simulink model "p1_MCU"  (R2023a)
settings: Solver=FixedStepDiscrete  StartTime=0.0  StopTime=inf  FixedStep=Ts_MCU  RelTol=1e-3  EnableMultiTasking=on
PreLoadFcn:
  | p1_params_new
  | spiDataDefinition
InitFcn:
  | mbd_s32k_consistency_checks(bdroot(gcs));
undefined symbols (not defined in the file or in its folder): ack, cpr_handwheel, cpr_steering, Discrete, DriverInput, DrivetrainLeft, DrivetrainRight, LQFP, MPU_IO, n_handwheel, n_steering, p1data, p1params, param, sr, steering_limit, SteeringLeft, SteeringRight, Time, Ts_MCU, wc, WheelForceLeft, WheelForceRight
libraries: simulink x74, mbd_s32k1xx_ec_toolbox x58, Library_Drivetrain x5, Library_Steering x5, etargetslib x3, ctrlSharedLib x1
(part 2 of 4)

== system p1_MCU/Subsystem ==
  ADC_Config : mbd_s32k1xx_ec_toolbox/Motor Control Blocks/ADC Blocks/ADC_Config  instance=0  mode=12-bit conversion  smplts=20  adiclk=alternate clock 1  adiv=input clock  show_adv_opts=on  pretrgsel=PDB pre-trigger  swpretrg=Disabled  adtrg=software  trgsel=TRGMUX output  refsel=Vrefh and Vrefl  supply_monitoring=off  acfe=off  acfgt=off  acren=off  cv1=0  cv2=0  adco=off  avge=off  avgs=4 samples
  ADC_Config1 : mbd_s32k1xx_ec_toolbox/Motor Control Blocks/ADC Blocks/ADC_Config  instance=1  mode=12-bit conversion  smplts=20  adiclk=alternate clock 1  adiv=input clock  show_adv_opts=on  pretrgsel=PDB pre-trigger  swpretrg=Disabled  adtrg=software  trgsel=TRGMUX output  refsel=Vrefh and Vrefl  supply_monitoring=off  acfe=off  acfgt=off  acren=off  cv1=0  cv2=0  adco=off  avge=off  avgs=4 samples
  Init Processor : mbd_s32k1xx_ec_toolbox/MBD_S32K1xx_Config_Information  mbdt_ver=0  disp_str=|  config_params=[]  mcu_target_name=S32K144  mcu_target_package=100-LQFP  mcu_target_sram_size=64KB  mcu_system_clock_freq=80  mcu_xtal_freq=External 8  mcu_steptick_timer=LPIT Channel 0  mcu_steptick_prio=15  ds_import_enable=on  target_compiler=GCC  target_memory=FLASH  gcc_target_compile_opts=-mcpu=cortex-m4 -mthumb -mfloat-abi=hard -mfpu=fpv4-sp-d16 -O1 -g -gstrict-dwarf  gcc_target_assemble_opts=-mcpu=cortex-m4 -mthumb -mfloat-abi=hard -mfpu=fpv4-sp-d16 -g  gcc_target_link_opts=-mcpu=cortex-m4 -mthumb -mfloat-abi=hard -mfpu=fpv4-sp-d16  gcc_target_default_lcf=on  gcc_target_user_lcf=S32K148_192_flash.ld  ghs_target_compile_opts=-cpu=cortexm4f -thumb -DARM_MATH_CM4 -fpu=vfpv4_d16 -fsingle -Ogeneral -Wundef -Wimplicit-int -Wshadow -Wtrigraphs --no_commons --gnu_asm -gnu99 -gdwarf-2 -G  ghs_target_assemble_opts=-cpu=cortexm4f -fpu=vfpv4_d16  ghs_target_link_opts=-cpu=cortexm4f -thumb -fpu=vfpv4_d16  ghs_target_default_lcf=on  ghs_target_user_lcf=S32K148_192_flash.ld  iar_target_compile_opts=--cpu=Cortex-M4F --thumb --fpu=VFPv4_sp -Ol -e --debug --dlib_config normal  iar_target_assemble_opts=--cpu Cortex-M4F --thumb --fpu VFPv4_sp  iar_target_link_opts=--no_exceptions --vfe --inline  iar_target_default_lcf=on  iar_target_user_lcf=S32K148_192_flash.icf  pil_download_enable=off  rbl_download_enable=off  rbl_start_delay=5000000  rbl_download_interface=OpenSDA  rbl_restart_request=off  rbl_com_port=Custom  rbl_com_port_custom=COM1  pil_download_rate=57600  pil_opensda_drive=Custom  pil_opensda_drive_custom=D  pil_uart_instance=1  pil_uart_rx=PTC6: [LPUART1_RX | Receive]  pil_uart_tx=PTC7: [LPUART1_TX | Transmit]  FTM_PWM_PcrCheckEnDis=on  FTM_Input_Edge_Inputs_PcrCheckEnDis=on  FTM_Dual_Edge_Inputs_PcrCheckEnDis=on  FTM_Quadrature_Inputs_PcrCheckEnDis=on  FTM_Hall_Sensor_Inputs_PcrCheckEnDis=on  LPTMR_PcrCheckEnDis=on  PIT_PcrCheckEnDis=on  RTC_PcrCheckEnDis=on  FlexCAN_PcrCheckEnDis=on  LIN_PcrCheckEnDis=on  FlexIO_PcrCheckEnDis=on  LPI2C_PcrCheckEnDis=on  LPSPI_PcrCheckEnDis=on  LPUART_PcrCheckEnDis=on  CMP_PcrCheckEnDis=on  GPIO_OutputPcrCheckEnDis=on  GPIO_InputPcrCheckEnDis=on  SBC_PcrCheckEnDis=on  BMS_PcrCheckEnDis=on  AMMCLIB_PcrCheckEnDis=on  FM_PcrCheckEnDis=on  Profile_PcrCheckEnDis=on  ConfigParams_PcrCheckEnDis=on  ModelRef_PcrCheckEnDis=on  PDB0_PcrCheckEnDis=on  CSEc_PcrCheckEnDis=on  eDMA_PcrCheckEnDis=on  FLASH_PcrCheckEnDis=on  ADC_PcrCheckEnDis=on  WDOG_PcrCheckEnDis=on
      | Target : S32K144-64KB_SRAM
      | Package : 100-pin
      | System clock : 80 MHz
      | XTAL clock : External 8 MHz
      | Compiler : IAR
      | Target Type : FLASH
      | Download Code after build : off
      | Step Tick Interrupt Priority : 15
  Init_CAN0_500kbit : mbd_s32k1xx_ec_toolbox/Communication Blocks/CAN Blocks/FCAN_Config  Priority=1  can_instance=0  can_mode=Normal mode  can_max_num_mb=16  can_rx=PTB0: [CAN0_RX | CAN Rx channel]  can_tx=PTB1: [CAN0_TX | CAN Tx Channel]  show_adv_opts=off  can_clk_src=Peripheral clock  bitrate=500  bitrate_adv_opts=off  can_presdiv=7  can_rjw=3  can_pseg1=6  can_pseg2=3  can_propseg=7  can_cbt_presdiv=9  can_cbt_rjw=0  can_cbt_pseg1=3  can_cbt_pseg2=3  can_cbt_propseg=6  can_fd_enable=off  can_payload=8  can_rxfifo_enable=off  can_fifo_id_filter_extended=off  can_fifo_id_filter_remote=off  can_num_id_filters=8  can_fifo_id_format=A  can_fifo_id_filter={'0x0', '0x0', '0x0', '0x0', '0x0', '0x0', '0x0', '0x0'}  can_pn_enable=off  can_wakeup_match=off  can_wakeup_timeout=off  can_timeout_en=off  can_match_timeout=1  can_multiple_matches_en=off  can_num_matches=1  can_idfilter_extendedid=off  can_idfilter_remoteframe=off  can_idfilter_type=Match exact  can_idfilter_id1=0  can_idfilter_id2=0  can_payloadfilter_enable=on  can_payloadfilter_dlclow=0  can_payloadfilter_dlchigh=0  can_payloadfilter_type=Match exact  can_payloadfilter_payload1_b0=0  can_payloadfilter_payload1_b1=0  can_payloadfilter_payload1_b2=0  can_payloadfilter_payload1_b3=0  can_payloadfilter_payload1_b4=0  can_payloadfilter_payload1_b5=0  can_payloadfilter_payload1_b6=0  can_payloadfilter_payload1_b7=0  can_payloadfilter_payload2_b0=0  can_payloadfilter_payload2_b1=0  can_payloadfilter_payload2_b2=0  can_payloadfilter_payload2_b3=0  can_payloadfilter_payload2_b4=0  can_payloadfilter_payload2_b5=0  can_payloadfilter_payload2_b6=0  can_payloadfilter_payload2_b7=0
  Init_CAN1_500kbit1 : mbd_s32k1xx_ec_toolbox/Communication Blocks/CAN Blocks/FCAN_Config  Priority=1  can_instance=1  can_mode=Normal mode  can_max_num_mb=16  can_rx=PTA12: [CAN1_RX | CAN Rx channel]  can_tx=PTA13: [CAN1_TX | CAN Tx Channel]  show_adv_opts=off  can_clk_src=Peripheral clock  bitrate=500  bitrate_adv_opts=off  can_presdiv=7  can_rjw=3  can_pseg1=6  can_pseg2=3  can_propseg=7  can_cbt_presdiv=9  can_cbt_rjw=0  can_cbt_pseg1=3  can_cbt_pseg2=3  can_cbt_propseg=6  can_fd_enable=off  can_payload=8  can_rxfifo_enable=off  can_fifo_id_filter_extended=off  can_fifo_id_filter_remote=off  can_num_id_filters=8  can_fifo_id_format=A  can_fifo_id_filter={'0x0', '0x0', '0x0', '0x0', '0x0', '0x0', '0x0', '0x0'}  can_pn_enable=off  can_wakeup_match=off  can_wakeup_timeout=off  can_timeout_en=off  can_match_timeout=1  can_multiple_matches_en=off  can_num_matches=1  can_idfilter_extendedid=off  can_idfilter_remoteframe=off  can_idfilter_type=Match exact  can_idfilter_id1=0  can_idfilter_id2=0  can_payloadfilter_enable=on  can_payloadfilter_dlclow=0  can_payloadfilter_dlchigh=0  can_payloadfilter_type=Match exact  can_payloadfilter_payload1_b0=0  can_payloadfilter_payload1_b1=0  can_payloadfilter_payload1_b2=0  can_payloadfilter_payload1_b3=0  can_payloadfilter_payload1_b4=0  can_payloadfilter_payload1_b5=0  can_payloadfilter_payload1_b6=0  can_payloadfilter_payload1_b7=0  can_payloadfilter_payload2_b0=0  can_payloadfilter_payload2_b1=0  can_payloadfilter_payload2_b2=0  can_payloadfilter_payload2_b3=0  can_payloadfilter_payload2_b4=0  can_payloadfilter_payload2_b5=0  can_payloadfilter_payload2_b6=0  can_payloadfilter_payload2_b7=0
  Init_CAN1_500kbit2 : mbd_s32k1xx_ec_toolbox/Communication Blocks/CAN Blocks/FCAN_Config  Priority=1  can_instance=2  can_mode=Normal mode  can_max_num_mb=16  can_rx=PTC16: [CAN2_RX | CAN Rx channel]  can_tx=PTC17: [CAN2_TX | CAN Tx Channel]  show_adv_opts=off  can_clk_src=Peripheral clock  bitrate=500  bitrate_adv_opts=off  can_presdiv=7  can_rjw=3  can_pseg1=6  can_pseg2=3  can_propseg=7  can_cbt_presdiv=9  can_cbt_rjw=0  can_cbt_pseg1=3  can_cbt_pseg2=3  can_cbt_propseg=6  can_fd_enable=off  can_payload=8  can_rxfifo_enable=off  can_fifo_id_filter_extended=off  can_fifo_id_filter_remote=off  can_num_id_filters=8  can_fifo_id_format=A  can_fifo_id_filter={'0x0', '0x0', '0x0', '0x0', '0x0', '0x0', '0x0', '0x0'}  can_pn_enable=off  can_wakeup_match=off  can_wakeup_timeout=off  can_timeout_en=off  can_match_timeout=1  can_multiple_matches_en=off  can_num_matches=1  can_idfilter_extendedid=off  can_idfilter_remoteframe=off  can_idfilter_type=Match exact  can_idfilter_id1=0  can_idfilter_id2=0  can_payloadfilter_enable=on  can_payloadfilter_dlclow=0  can_payloadfilter_dlchigh=0  can_payloadfilter_type=Match exact  can_payloadfilter_payload1_b0=0  can_payloadfilter_payload1_b1=0  can_payloadfilter_payload1_b2=0  can_payloadfilter_payload1_b3=0  can_payloadfilter_payload1_b4=0  can_payloadfilter_payload1_b5=0  can_payloadfilter_payload1_b6=0  can_payloadfilter_payload1_b7=0  can_payloadfilter_payload2_b0=0  can_payloadfilter_payload2_b1=0  can_payloadfilter_payload2_b2=0  can_payloadfilter_payload2_b3=0  can_payloadfilter_payload2_b4=0  can_payloadfilter_payload2_b5=0  can_payloadfilter_payload2_b6=0  can_payloadfilter_payload2_b7=0
  "LPSPI_Config " : mbd_s32k1xx_ec_toolbox/Communication Blocks/SPI Blocks/LPSPI_Config   InstanceNumber=1  Role=Slave  BaudRate=10000  ShowAdvanced=on  sin=PTB15: [LPSPI1_SIN | LPSPI Serial Data Input]  sout=PTB16: [LPSPI1_SOUT | LPSPI Serial Data Output]  sck=PTB14: [LPSPI1_SCK | LPSPI Serial Clock I/O]  pcs0=None  pcs1=None  pcs2=None  pcs3=PTB17: [LPSPI1_PCS3 | Peripheral Chip Select 3]  CPHA=0  CPOL=1  BitOrder=MSB first  TransferSize=8  WhichPCS=0  PCSPol=ActiveLow  ContinuousTransfer=off
  System Start : Subsystem  mask(System Start){ShowInLibBrowser=0}
      mask prompts: ShowInLibBrowser "Simulink:masks:CustCodeMaskParam1_MP"
      settings: CopyFcn=cccopyfcn(gcb)  OpenFcn=ccopenfcn('System Start Function')
      mask Help: eval('feval(''rtwprivate'',''rtwhelpview'',''rtw_sys_start_block'')');
      mask Display: disp('System\nStart');
  WDOG_Config : mbd_s32k1xx_ec_toolbox/Core and System Blocks/WDOG Blocks/WDOG_Config  clk_source=LPO clock  window_enable=off  window_value=1000.000 milliseconds  timeout_value=1000.000 milliseconds  prescaler_enable=on  update_enable=off  int_enable=off  show_adv_opts=on

== system p1_MCU/Subsystem1 ==
  note: Watchdog Reset
  note: Power Management
  note: Read ignition pin
  note: Only care about
      | first 16 bits
  note: Ticks to mV scaling
  note: Read supply voltage
  note: Send if Ign on
  note: Send if Ign off
  note: Buzzer
  note: Logic (net effect)
      | If ignition pin goes low the power is held alive for specified delay time before shutting down.
      |
      | If the ignition is resumed before shutdown can occur, the process resets
  note: Hold power alive
  ADC_Start : mbd_s32k1xx_ec_toolbox/Motor Control Blocks/ADC Blocks/ADC_Start  instance=0  adc_r=A  adc_chan=PTA6: [ADC0_SE2 | ADC Single Ended Input]  aien=off  mcuTargetUpdate=on
  Constant2 : Constant  Value=hex2dec('aa')  OutDataTypeStr=uint8
  Constant3 : Constant  Value=hex2dec('bb')  OutDataTypeStr=uint8
  Constant4 : Constant  Value=0  OutDataTypeStr=single
  Constant5 : Constant  Value=0.5  OutDataTypeStr=single
  Constant6 : Constant  Value=0  OutDataTypeStr=single
  Constant7 : Constant  Value=0  OutDataTypeStr=uint8
  Constant8 : Constant  OutDataTypeStr=uint8
  Data Store Memory2 : DataStoreMemory  DataStoreName=BattVolt  ReadBeforeWriteMsg=warning  WriteAfterWriteMsg=warning  WriteAfterReadMsg=warning  InitialValue=[0]  ShowAdditionalParam=off  OutDataTypeStr=uint16
  Data Store Memory4 : DataStoreMemory  DataStoreName=IgnState  ReadBeforeWriteMsg=warning  WriteAfterWriteMsg=warning  WriteAfterReadMsg=warning  InitialValue=[170]  ShowAdditionalParam=off  OutDataTypeStr=uint8
  Data Store Read : DataStoreRead  DataStoreName=BuzzerBool  IndexOptions=Index vector (dialog)  Indices=1  OutputSizes=1
  Data Store Write : DataStoreWrite  DataStoreName=BattVolt  IndexOptions=Index vector (dialog)  Indices=1  OutputSizes=1
  Data Store Write3 : DataStoreWrite  DataStoreName=IgnState  IndexOptions=Index vector (dialog)  Indices=1  OutputSizes=1
  Delay : Delay  DelayLength=1  InitialCondition=0
  Digital_Input : mbd_s32k1xx_ec_toolbox/GPIO Blocks/Digital_Input  gpio_pin=PTE13: [PTE13 | Port E I/O]  pull_resistor=Pulldown  passive_filter=off
  Digital_Output2 : mbd_s32k1xx_ec_toolbox/GPIO Blocks/Digital_Output  gpio_pin=PTD7: [PTD7 | Port D I/O]  init_val=High  drive_strength=Low
  Extract Bits : simulink/Logic and Bit Operations/Extract Bits  bitsToExtract=Lower half  numBits=8  bitIdxRange=[0 7]  outScalingMode=Treat bit field as an integer
  FTM_PWM_Config : mbd_s32k1xx_ec_toolbox/Motor Control Blocks/FTM Blocks/FTM_PWM_Config  ftmModule=2  ftmMode=Edge-Aligned PWM  ftmSourceClock=80 MHz  swcontrol_enable=off  chan0En=off  chan0Type=Complementary  chan2En=on  chan2Type=Independent  chan4En=off  chan4Type=Independent  chan6En=off  chan6Type=Independent  ftmPwmUnits=Hz  outFrequency=4000  ftmPeriod=20000  ftmPrescaler=Divide by 1  deadtimeUnits=Nanoseconds  deadtimeNs=0  deadtimeTicks=0  deadtimePrescaler=Divide by 1  dutyCycleCh0=0.25  dutyCycleCh1=0.25  dutyCycleCh2=0  dutyCycleCh3=0.5  dutyCycleCh4=0.25  dutyCycleCh5=0.25  dutyCycleCh6=0.25  dutyCycleCh7=0.25  dutyCycleSim=off  startAfterInit=on  showAdvOpt=on  pinFtmCh0=PTC5: [FTM2_CH0 | FTM Channel]  pinFtmCh1=None  pinPolCh0=Active Low  pinPolCh1=Active Low  outputComplem0=Main duplicated  outputLevel0=Low  outputLevel1=Low  pinFtmCh2=PTE4: [FTM2_CH2 | FTM Channel]  pinFtmCh3=PTD5: [FTM2_CH3 | FTM Channel]  pinPolCh2=Active Low  pinPolCh3=Active High  outputComplem2=Main duplicated  outputLevel2=High  outputLevel3=Low  pinFtmCh4=PTD13: [FTM2_CH4 | FTM Channel]  pinFtmCh5=None  pinPolCh4=Active Low  pinPolCh5=Active Low  outputComplem4=Main duplicated  outputLevel4=Low  outputLevel5=Low  pinFtmCh6=PTC12: [FTM2_CH6 | FTM Channel]  pinFtmCh7=None  pinPolCh6=Active Low  pinPolCh7=Active Low  outputComplem6=Main duplicated  outputLevel6=Low  outputLevel7=Low  initTrigger=off  chTrigger0=off  chTrigger1=off  chTrigger2=off  chTrigger3=off  chTrigger4=off  chTrigger5=off  chTrigger6=off  chTrigger7=off  mcuTargetUpdate=on  pwmSyncTrg=Software trigger  pwmSyncHwRouting=TRGMUX_FTM7  pwmSyncTrg0=off  pwmSyncTrg1=off  pwmSyncTrg2=off  pwmSyncAutoClear=on  pwmSyncMinLoad=on  pwmSyncMaxLoad=on  pwmSyncInvert=System Clock  pwmSyncOutControl=System Clock  pwmSyncOutMask=System Clock  pwmSyncCounterInitial=System Clock  pwmSyncPoints=Update now  reloadEnable=off  reloadPriority=15  reloadHalfCycle=off  reloadHCR=0  reloadFrequency=0  chnMatch0=off  chnMatch1=off  chnMatch2=off  chnMatch3=off  chnMatch4=off  chnMatch5=off  chnMatch6=off  chnMatch7=off  pwmFaultProtection=off  pwmFaultInterrupt=off  pwmFaultClearing=Fault control disabled  pwmFaultPinState=Safe Value  pwmFaultFilterValue=0  pwmFaultPriority=15  fault_disen_0=off  fault_filter_0=off  fault_polarity_0=Active High  fault_disen_1=off  fault_filter_1=off  fault_polarity_1=Active high  fault_disen_2=off  fault_filter_2=off  fault_polarity_2=Active high  fault_disen_3=off  fault_filter_3=off  fault_polarity_3=Active high  fault_pin_0=None  fault_pin_1=None  fault_pin_2=None  fault_pin_3=None
  Gain : Gain  Gain=9.5  OutDataTypeStr=uint16
  Relational Operator : RelationalOperator  Operator=<  OutDataTypeStr=boolean  RndMeth=Simplest
  Shutdown Delay (s) : Constant  Value=10  OutDataTypeStr=uint32
  Sum : Sum
  Switch : Switch  Criteria=u2 > Threshold  SaturateOnIntegerOverflow=off  InputSameDT=off
  Switch1 : Switch  Criteria=u2 > Threshold  OutDataTypeStr=single  SaturateOnIntegerOverflow=off  InputSameDT=off
  Switch2 : Switch  Criteria=u2 > Threshold  OutDataTypeStr=uint32  SaturateOnIntegerOverflow=off  InputSameDT=off
  WDOG_Trigger : mbd_s32k1xx_ec_toolbox/Core and System Blocks/WDOG Blocks/WDOG_Trigger
  Weighted Sample Time : SampleTimeMath  TsampMathOp=/  OutDataTypeStr=Inherit: Inherit via back propagation  RndMeth=Round  SaturateOnIntegerOverflow=on
  piSPISend : Subsystem  TreatAsAtomicUnit=on
  wires:
  Constant3/1 -> Switch/3
  Constant2/1 -> Switch/1
  Extract Bits/1 -> Gain/1
  ADC_Start/1 -> Extract Bits/1
  Switch/1 -> Data Store Write3/1
  Data Store Read/1 -> Switch1/2  "On/off"
  Switch1/1 -> FTM_PWM_Config/2
  Constant5/1 -> Switch1/1
  Constant4/1 -> FTM_PWM_Config/1
  Constant6/1 -> Switch1/3
  Gain/1 -> Data Store Write/1
  Relational Operator/1 -> Digital_Output2/1
  Shutdown Delay (s)/1 -> Weighted Sample Time/1
  Weighted Sample Time/1 -> Relational Operator/2
  Switch2/1 -> Delay/1, Relational Operator/1
  Constant8/1 -> Sum/1
  Constant7/1 -> Switch2/1
  Digital_Input/1 -> Switch2/2, Switch/2  "Ignition"
  Sum/1 -> Switch2/3
  Delay/1 -> Sum/2

== system p1_MCU/Subsystem2 ==
  If : If  IfExpression=u1 == 0  ShowElse=off
  If Action Subsystem : Subsystem  TreatAsAtomicUnit=on
  Init Flag Memory : DataStoreMemory  DataStoreName=init_flag  ReadBeforeWriteMsg=warning  WriteAfterWriteMsg=warning  WriteAfterReadMsg=warning  ShowAdditionalParam=off  OutDataTypeStr=uint32
  Init Flag Read : DataStoreRead  DataStoreName=init_flag  IndexOptions=Index vector (dialog)  Indices=1  OutputSizes=1
  wires:
  Init Flag Read/1 -> If/1
  If/1 -> If Action Subsystem/Action

== system p1_MCU/WFT CAN Receive ==
  FCAN_Isr : mbd_s32k1xx_ec_toolbox/Communication Blocks/CAN Blocks/FCAN_Isr  can_instance=2  can_event=Rx Complete
  Function-Call Subsystem : Subsystem  TreatAsAtomicUnit=on
  Terminator : Terminator
  Terminator1 : Terminator
  wires:
  FCAN_Isr/6 -> Function-Call Subsystem/5(Time Stamp)
  FCAN_Isr/1 -> Function-Call Subsystem/Trigger
  FCAN_Isr/3 -> Function-Call Subsystem/2(MSG ID)
  FCAN_Isr/4 -> Function-Call Subsystem/3(Data Packet)
  FCAN_Isr/5 -> Function-Call Subsystem/4(Data Length)
  FCAN_Isr/2 -> Function-Call Subsystem/1(Message Buffer)
  Function-Call Subsystem/1(WFT Feedback Left) -> Terminator/1  "WFT Left"
  Function-Call Subsystem/2(WFT Feedback Right) -> Terminator1/1  "WFT Right"

== system p1_MCU/ Controls Data Reception/Function-Call Subsystem1 ==
  Raw Encoder Estimate : Inport
  Fused Angle Estimate : Inport  Port=2
  SimTime : Inport  Port=3
  function : TriggerPort  TriggerType=function-call  VariantControl=Variant
  If : If  IfExpression=u1 > 0.1  ShowElse=off
  If Action Subsystem : Subsystem  TreatAsAtomicUnit=on
  Latched Encoder Offset : Outport  InitialOutput=[0]
  Time of Latch : Outport  Port=2  InitialOutput=[0]
  wires:
  SimTime/1 -> If Action Subsystem/3(SimTime), If/1
  If/1 -> If Action Subsystem/Action
  If Action Subsystem/1(Latched Encoder Offset) -> Latched Encoder Offset/1
  Raw Encoder Estimate/1 -> If Action Subsystem/1(Raw Encoder Estimate)
  Fused Angle Estimate/1 -> If Action Subsystem/2(Fused Angle Estimate)
  If Action Subsystem/2(Time of Latch) -> Time of Latch/1

== system p1_MCU/ Controls Data Reception/HW Encoder Reception ==
  AND : Logic  IconShape=distinctive  AllPortsSameDT=off  OutDataTypeStr=boolean
  AND1 : Logic  IconShape=distinctive  AllPortsSameDT=off  OutDataTypeStr=boolean
  Add : Sum  Inputs=+++  InputSameDT=on
  Add1 : Sum  InputSameDT=on  AccumDataTypeStr=int32  OutDataTypeStr=int32  SaturateOnIntegerOverflow=on
  Constant : Constant  Value=0  OutDataTypeStr=int32
  Constant1 : Constant  Value=65535  OutDataTypeStr=int32
  Constant2 : Constant  Value=-65535  OutDataTypeStr=int32
  Constant6 : Constant  Value=0  OutDataTypeStr=int32
  Data Type Conversion : DataTypeConversion  OutDataTypeStr=int32  SaturateOnIntegerOverflow=off  RndMeth=Floor
  Data Type Conversion1 : DataTypeConversion  OutDataTypeStr=int32  SaturateOnIntegerOverflow=off  RndMeth=Floor
  Memory : Memory  LinearizeAsDelay=on
  NOT : Logic  Operator=NOT  IconShape=distinctive  AllPortsSameDT=off  OutDataTypeStr=boolean
  Quadrature_Decoder : mbd_s32k1xx_ec_toolbox/Motor Control Blocks/FTM Blocks/Quadrature_Decoder  Priority=1  ftmModule=1  ec_mode=Phase A and Phase B  prescaler=1  cntin=0  mod=65535  phA_filtr_en=off  phA_filter=0  phA_pin=PTC7: [FTM1_QD_PHA | FTM quadrature Decode PhaseA]  polA=Normal  phB_filtr_en=off  phB_filter=0  phB_pin=PTC6: [FTM1_QD_PHB | FTM quadrature Decode PhaseB]  polB=Normal
  Switch : Switch  Criteria=u2 > Threshold  OutDataTypeStr=int32  SaturateOnIntegerOverflow=off
  Switch1 : Switch  Criteria=u2 > Threshold  OutDataTypeStr=int32  SaturateOnIntegerOverflow=off
  Terminator : Terminator
  HW Encoder Unwrapped : Outport
  HW Encoder : Outport  Port=2
  wires:
  Quadrature_Decoder/2 -> Terminator/1
  Quadrature_Decoder/3 -> AND1/1, AND/1
  Quadrature_Decoder/4 -> NOT/1, AND/2
  Quadrature_Decoder/1 -> Data Type Conversion/1  "Raw_HW_Encoder"
  Add/1 -> Memory/1, Add1/2
  AND/1 -> Switch/2
  Switch/1 -> Add/2
  Switch1/1 -> Add/3
  Constant/1 -> Switch/3
  Constant1/1 -> Switch/1
  Constant2/1 -> Switch1/1
  AND1/1 -> Switch1/2
  NOT/1 -> AND1/2
  Data Type Conversion/1 -> HW Encoder/1, Add1/1
  Memory/1 -> Add/1
  Constant6/1 -> Switch1/3
  Add1/1 -> Data Type Conversion1/1
  Data Type Conversion1/1 -> HW Encoder Unwrapped/1

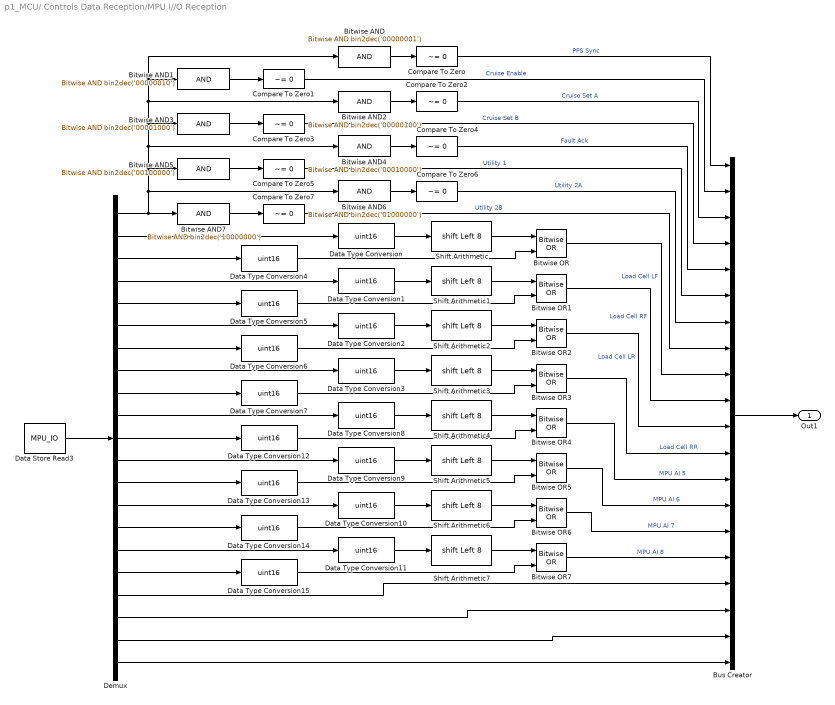
== system p1_MCU/ Controls Data Reception/MPU I//O Reception ==
  Bitwise AND : simulink/Logic and Bit Operations/Bitwise Operator  logicop=AND  UseBitMask=on  BitMask=bin2dec('00000001')  BitMaskRealWorld=Stored Integer
  Bitwise AND1 : simulink/Logic and Bit Operations/Bitwise Operator  logicop=AND  UseBitMask=on  BitMask=bin2dec('00000010')  BitMaskRealWorld=Stored Integer
  Bitwise AND2 : simulink/Logic and Bit Operations/Bitwise Operator  logicop=AND  UseBitMask=on  BitMask=bin2dec('00000100')  BitMaskRealWorld=Stored Integer
  Bitwise AND3 : simulink/Logic and Bit Operations/Bitwise Operator  logicop=AND  UseBitMask=on  BitMask=bin2dec('00001000')  BitMaskRealWorld=Stored Integer
  Bitwise AND4 : simulink/Logic and Bit Operations/Bitwise Operator  logicop=AND  UseBitMask=on  BitMask=bin2dec('00010000')  BitMaskRealWorld=Stored Integer
  Bitwise AND5 : simulink/Logic and Bit Operations/Bitwise Operator  logicop=AND  UseBitMask=on  BitMask=bin2dec('00100000')  BitMaskRealWorld=Stored Integer
  Bitwise AND6 : simulink/Logic and Bit Operations/Bitwise Operator  logicop=AND  UseBitMask=on  BitMask=bin2dec('01000000')  BitMaskRealWorld=Stored Integer
  Bitwise AND7 : simulink/Logic and Bit Operations/Bitwise Operator  logicop=AND  UseBitMask=on  BitMask=bin2dec('10000000')  BitMaskRealWorld=Stored Integer
  Bitwise OR{,1..7} (8 alike) : simulink/Logic and Bit Operations/Bitwise Operator  logicop=OR  UseBitMask=off  NumInputPorts=2  BitMask=bin2dec('11011001')  BitMaskRealWorld=Stored Integer
  Bus Creator : BusCreator  Inputs=20
  Compare To Zero{,1..7} (8 alike) : simulink/Logic and Bit Operations/Compare To Zero  relop=~=  OutDataTypeStr=boolean
  Data Store Read3 : DataStoreRead  DataStoreName=MPU_IO  IndexOptions=Index vector (dialog)  Indices=1  OutputSizes=1
  Data Type Conversion{,1..15} (16 alike) : DataTypeConversion  OutDataTypeStr=uint16  SaturateOnIntegerOverflow=off  RndMeth=Floor
  Demux : Demux  Outputs=21
  Shift Arithmetic{,1..7} (8 alike) : ArithShift  BitShiftNumber=8  BitShiftDirection=Left
  Out1 : Outport
  wires:
  Data Store Read3/1 -> Demux/1
  Bus Creator/1 -> Out1/1
  Bitwise AND/1 -> Compare To Zero/1
  Demux/1 -> Bitwise AND/1, Bitwise AND1/1, Bitwise AND2/1, Bitwise AND3/1, Bitwise AND4/1, Bitwise AND5/1, Bitwise AND6/1, Bitwise AND7/1
  Bitwise AND1/1 -> Compare To Zero1/1
  Bitwise AND2/1 -> Compare To Zero2/1
  Bitwise AND3/1 -> Compare To Zero3/1
  Bitwise AND7/1 -> Compare To Zero7/1
  Bitwise AND6/1 -> Compare To Zero6/1
  Bitwise AND5/1 -> Compare To Zero5/1
  Bitwise AND4/1 -> Compare To Zero4/1
  Demux/2 -> Data Type Conversion/1
  Data Type Conversion/1 -> Shift Arithmetic/1
  Demux/4 -> Data Type Conversion1/1
  Data Type Conversion1/1 -> Shift Arithmetic1/1
  Data Type Conversion2/1 -> Shift Arithmetic2/1
  Demux/6 -> Data Type Conversion2/1
  Data Type Conversion3/1 -> Shift Arithmetic3/1
  Demux/8 -> Data Type Conversion3/1
  Demux/3 -> Data Type Conversion4/1
  Demux/5 -> Data Type Conversion5/1
  Demux/7 -> Data Type Conversion6/1
  Demux/9 -> Data Type Conversion7/1
  Data Type Conversion4/1 -> Bitwise OR/2
  Shift Arithmetic/1 -> Bitwise OR/1
  Shift Arithmetic1/1 -> Bitwise OR1/1
  Shift Arithmetic2/1 -> Bitwise OR2/1
  Shift Arithmetic3/1 -> Bitwise OR3/1
  Data Type Conversion5/1 -> Bitwise OR1/2
  Data Type Conversion6/1 -> Bitwise OR2/2
  Data Type Conversion7/1 -> Bitwise OR3/2
  Compare To Zero/1 -> Bus Creator/1  "PPS Sync"
  Compare To Zero2/1 -> Bus Creator/3  "Cruise Set A"
  Compare To Zero4/1 -> Bus Creator/5  "Fault Ack"
  Compare To Zero6/1 -> Bus Creator/7  "Utility 2A"
  Compare To Zero7/1 -> Bus Creator/8  "Utility 2B"
  Compare To Zero5/1 -> Bus Creator/6  "Utility 1"
  Compare To Zero3/1 -> Bus Creator/4  "Cruise Set B"
  Compare To Zero1/1 -> Bus Creator/2  "Cruise Enable"
  Bitwise OR/1 -> Bus Creator/9  "Load Cell LF"
  Data Type Conversion12/1 -> Bitwise OR4/2
  Demux/14 -> Data Type Conversion10/1
  Demux/15 -> Data Type Conversion14/1
  Demux/16 -> Data Type Conversion11/1
  Demux/12 -> Data Type Conversion9/1
  Demux/10 -> Data Type Conversion8/1
  Demux/11 -> Data Type Conversion12/1
  Demux/13 -> Data Type Conversion13/1
  Demux/17 -> Data Type Conversion15/1
  Shift Arithmetic6/1 -> Bitwise OR6/1
  Data Type Conversion15/1 -> Bitwise OR7/2
  Data Type Conversion10/1 -> Shift Arithmetic6/1
  Shift Arithmetic4/1 -> Bitwise OR4/1
  Data Type Conversion13/1 -> Bitwise OR5/2
  Shift Arithmetic5/1 -> Bitwise OR5/1
  Shift Arithmetic7/1 -> Bitwise OR7/1
  Data Type Conversion8/1 -> Shift Arithmetic4/1
  Data Type Conversion9/1 -> Shift Arithmetic5/1
  Data Type Conversion11/1 -> Shift Arithmetic7/1
  Data Type Conversion14/1 -> Bitwise OR6/2
  Bitwise OR1/1 -> Bus Creator/10  "Load Cell RF"
  Bitwise OR2/1 -> Bus Creator/11  "Load Cell LR"
  Bitwise OR3/1 -> Bus Creator/12  "Load Cell RR"
  Bitwise OR4/1 -> Bus Creator/13  "MPU AI 5"
  Bitwise OR5/1 -> Bus Creator/14  "MPU AI 6"
  Bitwise OR6/1 -> Bus Creator/15  "MPU AI 7"
  Bitwise OR7/1 -> Bus Creator/16  "MPU AI 8"
  Demux/21 -> Bus Creator/20
  Demux/20 -> Bus Creator/19
  Demux/19 -> Bus Creator/18
  Demux/18 -> Bus Creator/17

== system p1_MCU/ Controls Data Reception/P1_Byte_Pack ==
  In1 : Inport
  Bitwise AND : simulink/Logic and Bit Operations/Bitwise Operator  logicop=AND  UseBitMask=on  BitMask=hex2dec('000000FF')  BitMaskRealWorld=Stored Integer
  Bitwise AND1 : simulink/Logic and Bit Operations/Bitwise Operator  logicop=AND  UseBitMask=on  BitMask=hex2dec('0000FF00')  BitMaskRealWorld=Stored Integer
  Bitwise AND2 : simulink/Logic and Bit Operations/Bitwise Operator  logicop=AND  UseBitMask=on  BitMask=hex2dec('00FF0000')  BitMaskRealWorld=Stored Integer
  Bitwise AND3 : simulink/Logic and Bit Operations/Bitwise Operator  logicop=AND  UseBitMask=on  BitMask=hex2dec('FF000000')  BitMaskRealWorld=Stored Integer
  Data Type Conversion{,1..3} (4 alike) : DataTypeConversion  OutDataTypeStr=uint8  ConvertRealWorld=Stored Integer (SI)  SaturateOnIntegerOverflow=off  RndMeth=Floor
  Data Type Conversion5 : DataTypeConversion  OutDataTypeStr=single  SaturateOnIntegerOverflow=off  RndMeth=Floor
  Float Typecast : FloatTypecast
  Mux : Mux
  Shift Arithmetic : ArithShift  BitShiftNumber=8  BitShiftDirection=Right
  Shift Arithmetic1 : ArithShift  BitShiftNumber=16  BitShiftDirection=Right
  Shift Arithmetic2 : ArithShift  BitShiftNumber=24  BitShiftDirection=Right
  Out1 : Outport
  wires:
  Data Type Conversion3/1 -> Mux/4
  Data Type Conversion2/1 -> Mux/3
  Data Type Conversion1/1 -> Mux/2
  Data Type Conversion/1 -> Mux/1
  Bitwise AND/1 -> Data Type Conversion/1
  In1/1 -> Data Type Conversion5/1
  Mux/1 -> Out1/1
  Data Type Conversion5/1 -> Float Typecast/1
  Bitwise AND1/1 -> Shift Arithmetic/1
  Bitwise AND2/1 -> Shift Arithmetic1/1
  Bitwise AND3/1 -> Shift Arithmetic2/1
  Float Typecast/1 -> Bitwise AND3/1, Bitwise AND2/1, Bitwise AND/1, Bitwise AND1/1
  Shift Arithmetic/1 -> Data Type Conversion1/1
  Shift Arithmetic1/1 -> Data Type Conversion2/1
  Shift Arithmetic2/1 -> Data Type Conversion3/1

== system p1_MCU/ Controls Data Reception/P1_Byte_Pack1 ==
  In1 : Inport
  Bitwise AND : simulink/Logic and Bit Operations/Bitwise Operator  logicop=AND  UseBitMask=on  BitMask=hex2dec('000000FF')  BitMaskRealWorld=Stored Integer
  Bitwise AND1 : simulink/Logic and Bit Operations/Bitwise Operator  logicop=AND  UseBitMask=on  BitMask=hex2dec('0000FF00')  BitMaskRealWorld=Stored Integer
  Bitwise AND2 : simulink/Logic and Bit Operations/Bitwise Operator  logicop=AND  UseBitMask=on  BitMask=hex2dec('00FF0000')  BitMaskRealWorld=Stored Integer
  Bitwise AND3 : simulink/Logic and Bit Operations/Bitwise Operator  logicop=AND  UseBitMask=on  BitMask=hex2dec('FF000000')  BitMaskRealWorld=Stored Integer
  Data Type Conversion{,1..3} (4 alike) : DataTypeConversion  OutDataTypeStr=uint8  ConvertRealWorld=Stored Integer (SI)  SaturateOnIntegerOverflow=off  RndMeth=Floor
  Data Type Conversion5 : DataTypeConversion  OutDataTypeStr=single  SaturateOnIntegerOverflow=off  RndMeth=Floor
  Float Typecast : FloatTypecast
  Mux : Mux
  Shift Arithmetic : ArithShift  BitShiftNumber=8  BitShiftDirection=Right
  Shift Arithmetic1 : ArithShift  BitShiftNumber=16  BitShiftDirection=Right
  Shift Arithmetic2 : ArithShift  BitShiftNumber=24  BitShiftDirection=Right
  Out1 : Outport
  wires:
  Data Type Conversion3/1 -> Mux/4
  Data Type Conversion2/1 -> Mux/3
  Data Type Conversion1/1 -> Mux/2
  Data Type Conversion/1 -> Mux/1
  Bitwise AND/1 -> Data Type Conversion/1
  In1/1 -> Data Type Conversion5/1
  Mux/1 -> Out1/1
  Data Type Conversion5/1 -> Float Typecast/1
  Bitwise AND1/1 -> Shift Arithmetic/1
  Bitwise AND2/1 -> Shift Arithmetic1/1
  Bitwise AND3/1 -> Shift Arithmetic2/1
  Float Typecast/1 -> Bitwise AND3/1, Bitwise AND2/1, Bitwise AND/1, Bitwise AND1/1
  Shift Arithmetic/1 -> Data Type Conversion1/1
  Shift Arithmetic1/1 -> Data Type Conversion2/1
  Shift Arithmetic2/1 -> Data Type Conversion3/1

== system p1_MCU/ Controls Data Reception/P1_Byte_Pack2 ==
  Latched Encoder Offset : Inport
  Bitwise AND : simulink/Logic and Bit Operations/Bitwise Operator  logicop=AND  UseBitMask=on  BitMask=hex2dec('000000FF')  BitMaskRealWorld=Stored Integer
  Bitwise AND1 : simulink/Logic and Bit Operations/Bitwise Operator  logicop=AND  UseBitMask=on  BitMask=hex2dec('0000FF00')  BitMaskRealWorld=Stored Integer
  Bitwise AND2 : simulink/Logic and Bit Operations/Bitwise Operator  logicop=AND  UseBitMask=on  BitMask=hex2dec('00FF0000')  BitMaskRealWorld=Stored Integer
  Bitwise AND3 : simulink/Logic and Bit Operations/Bitwise Operator  logicop=AND  UseBitMask=on  BitMask=hex2dec('FF000000')  BitMaskRealWorld=Stored Integer
  Data Type Conversion{,1..3} (4 alike) : DataTypeConversion  OutDataTypeStr=uint8  ConvertRealWorld=Stored Integer (SI)  SaturateOnIntegerOverflow=off  RndMeth=Floor
  Data Type Conversion5 : DataTypeConversion  OutDataTypeStr=single  SaturateOnIntegerOverflow=off  RndMeth=Floor
  Float Typecast : FloatTypecast
  Mux : Mux
  Shift Arithmetic : ArithShift  BitShiftNumber=8  BitShiftDirection=Right
  Shift Arithmetic1 : ArithShift  BitShiftNumber=16  BitShiftDirection=Right
  Shift Arithmetic2 : ArithShift  BitShiftNumber=24  BitShiftDirection=Right
  Out1 : Outport
  wires:
  Shift Arithmetic2/1 -> Data Type Conversion3/1
  Shift Arithmetic1/1 -> Data Type Conversion2/1
  Shift Arithmetic/1 -> Data Type Conversion1/1
  Float Typecast/1 -> Bitwise AND1/1, Bitwise AND/1, Bitwise AND2/1, Bitwise AND3/1
  Bitwise AND3/1 -> Shift Arithmetic2/1
  Bitwise AND2/1 -> Shift Arithmetic1/1
  Bitwise AND1/1 -> Shift Arithmetic/1
  Data Type Conversion5/1 -> Float Typecast/1
  Mux/1 -> Out1/1
  Latched Encoder Offset/1 -> Data Type Conversion5/1
  Bitwise AND/1 -> Data Type Conversion/1
  Data Type Conversion/1 -> Mux/1
  Data Type Conversion1/1 -> Mux/2
  Data Type Conversion2/1 -> Mux/3
  Data Type Conversion3/1 -> Mux/4

== system p1_MCU/ Controls Data Reception/Subsystem ==
  In2 : Inport
  In1 : Inport  Port=2
  In3 : Inport  Port=3
  Add : Sum  Inputs=+++
  Data Type Conversion : DataTypeConversion  OutDataTypeStr=uint8  SaturateOnIntegerOverflow=off  RndMeth=Floor
  Data Type Conversion1 : DataTypeConversion  OutDataTypeStr=uint8  SaturateOnIntegerOverflow=off  RndMeth=Floor
  Data Type Conversion2 : DataTypeConversion  OutDataTypeStr=uint8  SaturateOnIntegerOverflow=off  RndMeth=Floor
  Gain : Gain  OutDataTypeStr=uint8  SaturateOnIntegerOverflow=on
  Gain1 : Gain  Gain=2  OutDataTypeStr=uint8  SaturateOnIntegerOverflow=on
  Gain2 : Gain  Gain=4  OutDataTypeStr=uint8  SaturateOnIntegerOverflow=on
  Out1 : Outport
  wires:
  In1/1 -> Data Type Conversion/1
  In2/1 -> Data Type Conversion1/1
  In3/1 -> Data Type Conversion2/1
  Add/1 -> Out1/1
  Gain/1 -> Add/1
  Gain1/1 -> Add/2
  Gain2/1 -> Add/3
  Data Type Conversion/1 -> Gain/1
  Data Type Conversion1/1 -> Gain1/1
  Data Type Conversion2/1 -> Gain2/1

== system p1_MCU/Drivetrain Management/Subsystem ==
  Driver Controls : Inport
  Torque Request : Inport  Port=2
  Pos Velocity Lim : Inport  Port=3
  Neg Velocity Lim : Inport  Port=4
  Steering Mode : Inport  Port=5
  Comms Good (Opposing Motor) : Inport  Port=6
  Vehicle Speed : Inport  Port=7
  Motor Feedback : Inport  Port=8
  Last CAN Time : Inport  Port=9
  Data Store Memory : DataStoreMemory  DataStoreName=param_CANTimeOut  ReadBeforeWriteMsg=warning  WriteAfterWriteMsg=warning  WriteAfterReadMsg=warning  InitialValue=p1params.drivetrain.left.CANTimeOut  ShowAdditionalParam=off  OutDataTypeStr=double
  Data Store Memory10 : DataStoreMemory  DataStoreName=param_minTorqueFullDrive  ReadBeforeWriteMsg=warning  WriteAfterWriteMsg=warning  WriteAfterReadMsg=warning  InitialValue=p1params.drivetrain.left.minTorqueFullDrive  ShowAdditionalParam=off  OutDataTypeStr=double
  Data Store Memory11 : DataStoreMemory  DataStoreName=param_maxTorqueFullDrive  ReadBeforeWriteMsg=warning  WriteAfterWriteMsg=warning  WriteAfterReadMsg=warning  InitialValue=p1params.drivetrain.left.maxTorqueFullDrive  ShowAdditionalParam=off  OutDataTypeStr=double
  Data Store Memory12 : DataStoreMemory  DataStoreName=fault_reset  ReadBeforeWriteMsg=warning  WriteAfterWriteMsg=warning  WriteAfterReadMsg=warning  ShowAdditionalParam=off  OutDataTypeStr=double
  Data Store Memory13 : DataStoreMemory  DataStoreName=fault_reason  ReadBeforeWriteMsg=warning  WriteAfterWriteMsg=warning  WriteAfterReadMsg=warning  ShowAdditionalParam=off  OutDataTypeStr=double
  Data Store Memory14 : DataStoreMemory  DataStoreName=param_AccelMaxV  ReadBeforeWriteMsg=warning  WriteAfterWriteMsg=warning  WriteAfterReadMsg=warning  InitialValue=p1params.input.VhighGuard  ShowAdditionalParam=off  OutDataTypeStr=double
  Data Store Memory3 : DataStoreMemory  DataStoreName=param_TorqueLimHigh  ReadBeforeWriteMsg=warning  WriteAfterWriteMsg=warning  WriteAfterReadMsg=warning  InitialValue=p1params.drivetrain.left.torqueLimHigh  ShowAdditionalParam=off  OutDataTypeStr=double
  Data Store Memory4 : DataStoreMemory  DataStoreName=param_TorqueLimLow  ReadBeforeWriteMsg=warning  WriteAfterWriteMsg=warning  WriteAfterReadMsg=warning  InitialValue=p1params.drivetrain.left.torqueLimLow  ShowAdditionalParam=off  OutDataTypeStr=double
  Data Store Memory5 : DataStoreMemory  DataStoreName=param_AccelMinV  ReadBeforeWriteMsg=warning  WriteAfterWriteMsg=warning  WriteAfterReadMsg=warning  InitialValue=p1params.input.VlowGuard  ShowAdditionalParam=off  OutDataTypeStr=double
  Data Store Memory7 : DataStoreMemory  DataStoreName=param_ZeroSpeedThresh  ReadBeforeWriteMsg=warning  WriteAfterWriteMsg=warning  WriteAfterReadMsg=warning  InitialValue=p1params.drivetrain.left.zeroSpeedThresh  ShowAdditionalParam=off  OutDataTypeStr=double
  Data Store Memory8 : DataStoreMemory  DataStoreName=param_minTorqueStartDrive  ReadBeforeWriteMsg=warning  WriteAfterWriteMsg=warning  WriteAfterReadMsg=warning  InitialValue=p1params.drivetrain.left.minTorqueStartDrive  ShowAdditionalParam=off  OutDataTypeStr=double
  Data Store Memory9 : DataStoreMemory  DataStoreName=param_maxTorqueStartDrive  ReadBeforeWriteMsg=warning  WriteAfterWriteMsg=warning  WriteAfterReadMsg=warning  InitialValue=p1params.drivetrain.left.maxTorqueStartDrive  ShowAdditionalParam=off  OutDataTypeStr=double
  Data Store Write : DataStoreWrite  DataStoreName=DrivetrainLeft  DataStoreElements=DrivetrainLeft(1)  IndexOptions=Index vector (dialog)  Indices=1  OutputSizes=1
  Data Store Write1 : DataStoreWrite  DataStoreName=DrivetrainLeft  DataStoreElements=DrivetrainLeft(3:10)  IndexOptions=Index vector (dialog)  Indices=1  OutputSizes=1
  UQM Control Logic : Library_Drivetrain/UQM Control Logic  SystemSampleTime=-1  VariantActivationTime=update diagram  Latency=0  AutoFrameSizeCalculation=off
  Drive Fault Lamp : Outport
  Universal Command : Outport  Port=2
  Comms Good Flag : Outport  Port=3
  wires:
  Driver Controls/1 -> UQM Control Logic/1
  Torque Request/1 -> UQM Control Logic/2
  Pos Velocity Lim/1 -> UQM Control Logic/3
  Neg Velocity Lim/1 -> UQM Control Logic/4
  Steering Mode/1 -> UQM Control Logic/5
  Comms Good (Opposing Motor)/1 -> UQM Control Logic/6
  Vehicle Speed/1 -> UQM Control Logic/7
  Motor Feedback/1 -> UQM Control Logic/8
  UQM Control Logic/2 -> Drive Fault Lamp/1
  UQM Control Logic/1 -> Data Store Write/1
  UQM Control Logic/3 -> Data Store Write1/1, Universal Command/1
  UQM Control Logic/4 -> Comms Good Flag/1
  Last CAN Time/1 -> UQM Control Logic/9

== system p1_MCU/Drivetrain Management/Subsystem1 ==
  Driver Controls : Inport
  Torque Request : Inport  Port=2
  Pos Velocity Lim : Inport  Port=3
  Neg Velocity Lim : Inport  Port=4
  Steering Mode : Inport  Port=5
  Comms Good (Opposing Motor) : Inport  Port=6
  Vehicle Speed : Inport  Port=7
  Motor Feedback : Inport  Port=8
  Last CAN Time : Inport  Port=9
  Data Store Memory : DataStoreMemory  DataStoreName=param_CANTimeOut  ReadBeforeWriteMsg=warning  WriteAfterWriteMsg=warning  WriteAfterReadMsg=warning  InitialValue=p1params.drivetrain.right.CANTimeOut  ShowAdditionalParam=off  OutDataTypeStr=double
  Data Store Memory1 : DataStoreMemory  DataStoreName=param_VelLimFWD  ReadBeforeWriteMsg=warning  WriteAfterWriteMsg=warning  WriteAfterReadMsg=warning  InitialValue=p1params.drivetrain.right.velLimFWD  ShowAdditionalParam=off  OutDataTypeStr=double
  Data Store Memory10 : DataStoreMemory  DataStoreName=param_minTorqueFullDrive  ReadBeforeWriteMsg=warning  WriteAfterWriteMsg=warning  WriteAfterReadMsg=warning  InitialValue=p1params.drivetrain.right.minTorqueFullDrive  ShowAdditionalParam=off  OutDataTypeStr=double
  Data Store Memory11 : DataStoreMemory  DataStoreName=param_maxTorqueFullDrive  ReadBeforeWriteMsg=warning  WriteAfterWriteMsg=warning  WriteAfterReadMsg=warning  InitialValue=p1params.drivetrain.right.maxTorqueFullDrive  ShowAdditionalParam=off  OutDataTypeStr=double
  Data Store Memory12 : DataStoreMemory  DataStoreName=fault_reset  ReadBeforeWriteMsg=warning  WriteAfterWriteMsg=warning  WriteAfterReadMsg=warning  ShowAdditionalParam=off  OutDataTypeStr=double
  Data Store Memory13 : DataStoreMemory  DataStoreName=fault_reason  ReadBeforeWriteMsg=warning  WriteAfterWriteMsg=warning  WriteAfterReadMsg=warning  ShowAdditionalParam=off  OutDataTypeStr=double
  Data Store Memory2 : DataStoreMemory  DataStoreName=param_VelLimREV  ReadBeforeWriteMsg=warning  WriteAfterWriteMsg=warning  WriteAfterReadMsg=warning  InitialValue=p1params.drivetrain.right.velLimREV  ShowAdditionalParam=off  OutDataTypeStr=double
  Data Store Memory3 : DataStoreMemory  DataStoreName=param_TorqueLimHigh  ReadBeforeWriteMsg=warning  WriteAfterWriteMsg=warning  WriteAfterReadMsg=warning  InitialValue=p1params.drivetrain.right.torqueLimHigh  ShowAdditionalParam=off  OutDataTypeStr=double
  Data Store Memory4 : DataStoreMemory  DataStoreName=param_TorqueLimLow  ReadBeforeWriteMsg=warning  WriteAfterWriteMsg=warning  WriteAfterReadMsg=warning  InitialValue=p1params.drivetrain.right.torqueLimLow  ShowAdditionalParam=off  OutDataTypeStr=double
  Data Store Memory5 : DataStoreMemory  DataStoreName=param_AccelMinV  ReadBeforeWriteMsg=warning  WriteAfterWriteMsg=warning  WriteAfterReadMsg=warning  InitialValue=p1params.input.VlowGuard  ShowAdditionalParam=off  OutDataTypeStr=double
  Data Store Memory6 : DataStoreMemory  DataStoreName=param_AccelMaxV  ReadBeforeWriteMsg=warning  WriteAfterWriteMsg=warning  WriteAfterReadMsg=warning  InitialValue=p1params.input.VhighGuard  ShowAdditionalParam=off  OutDataTypeStr=double
  Data Store Memory7 : DataStoreMemory  DataStoreName=param_ZeroSpeedThresh  ReadBeforeWriteMsg=warning  WriteAfterWriteMsg=warning  WriteAfterReadMsg=warning  InitialValue=p1params.drivetrain.right.zeroSpeedThresh  ShowAdditionalParam=off  OutDataTypeStr=double
  Data Store Memory8 : DataStoreMemory  DataStoreName=param_minTorqueStartDrive  ReadBeforeWriteMsg=warning  WriteAfterWriteMsg=warning  WriteAfterReadMsg=warning  InitialValue=p1params.drivetrain.right.minTorqueStartDrive  ShowAdditionalParam=off  OutDataTypeStr=double
  Data Store Memory9 : DataStoreMemory  DataStoreName=param_maxTorqueStartDrive  ReadBeforeWriteMsg=warning  WriteAfterWriteMsg=warning  WriteAfterReadMsg=warning  InitialValue=p1params.drivetrain.right.maxTorqueStartDrive  ShowAdditionalParam=off  OutDataTypeStr=double
  Data Store Write : DataStoreWrite  DataStoreName=DrivetrainRight  DataStoreElements=DrivetrainRight(1)  IndexOptions=Index vector (dialog)  Indices=1  OutputSizes=1
  Data Store Write1 : DataStoreWrite  DataStoreName=DrivetrainRight  DataStoreElements=DrivetrainRight(3:10)  IndexOptions=Index vector (dialog)  Indices=1  OutputSizes=1
  UQM Control Logic (R) : Library_Drivetrain/UQM Control Logic  SystemSampleTime=-1  VariantActivationTime=update diagram  Latency=0  AutoFrameSizeCalculation=off
  Drive Fault Lamp : Outport
  Universal Command : Outport  Port=2
  Comms Good Flag : Outport  Port=3
  wires:
  Driver Controls/1 -> UQM Control Logic (R)/1
  Torque Request/1 -> UQM Control Logic (R)/2
  Pos Velocity Lim/1 -> UQM Control Logic (R)/3
  Neg Velocity Lim/1 -> UQM Control Logic (R)/4
  Steering Mode/1 -> UQM Control Logic (R)/5
  Comms Good (Opposing Motor)/1 -> UQM Control Logic (R)/6
  Vehicle Speed/1 -> UQM Control Logic (R)/7
  Motor Feedback/1 -> UQM Control Logic (R)/8
  UQM Control Logic (R)/2 -> Drive Fault Lamp/1
  UQM Control Logic (R)/1 -> Data Store Write/1
  UQM Control Logic (R)/3 -> Data Store Write1/1, Universal Command/1
  UQM Control Logic (R)/4 -> Comms Good Flag/1
  Last CAN Time/1 -> UQM Control Logic (R)/9

== system p1_MCU/Driving Controls Indicators/Subsystem ==
  Forward : Inport
  Reverse : Inport  Port=2
  GPS OK : Inport  Port=3
  WFT OK : Inport  Port=4
  Drive Fault : Inport  Port=5
  Steer Fault : Inport  Port=6
  Add : Sum  Inputs=++++++
  Data Type Conversion{,1..5} (6 alike) : DataTypeConversion  OutDataTypeStr=uint8  SaturateOnIntegerOverflow=off  RndMeth=Floor
  Gain : Gain  OutDataTypeStr=uint8  SaturateOnIntegerOverflow=on
  Gain1 : Gain  Gain=2  OutDataTypeStr=uint8  SaturateOnIntegerOverflow=on
  Gain2 : Gain  Gain=4  OutDataTypeStr=uint8  SaturateOnIntegerOverflow=on
  Gain3 : Gain  Gain=8  OutDataTypeStr=uint8  SaturateOnIntegerOverflow=on
  Gain4 : Gain  Gain=16  OutDataTypeStr=uint8  SaturateOnIntegerOverflow=on
  Gain5 : Gain  Gain=32  OutDataTypeStr=uint8  SaturateOnIntegerOverflow=on
  Out1 : Outport
  wires:
  Forward/1 -> Data Type Conversion/1
  Reverse/1 -> Data Type Conversion1/1
  GPS OK/1 -> Data Type Conversion2/1
  Add/1 -> Out1/1
  Gain/1 -> Add/1
  Gain1/1 -> Add/2
  Gain2/1 -> Add/3
  Data Type Conversion/1 -> Gain/1
  Data Type Conversion1/1 -> Gain1/1
  Data Type Conversion2/1 -> Gain2/1
  Steer Fault/1 -> Data Type Conversion5/1
  Data Type Conversion3/1 -> Gain3/1
  Gain5/1 -> Add/6
  WFT OK/1 -> Data Type Conversion3/1
  Data Type Conversion4/1 -> Gain4/1
  Data Type Conversion5/1 -> Gain5/1
  Drive Fault/1 -> Data Type Conversion4/1
  Gain3/1 -> Add/4
  Gain4/1 -> Add/5

== system p1_MCU/Driving Controls Indicators/Subsystem1 ==
  Cruise Enable : Inport
  Cruise Active : Inport  Port=2
  Fault Ack : Inport  Port=3
  Utility 1 : Inport  Port=4
  Add : Sum  Inputs=++++
  Data Type Conversion{,1..3} (4 alike) : DataTypeConversion  OutDataTypeStr=uint8  SaturateOnIntegerOverflow=off  RndMeth=Floor
  Gain : Gain  OutDataTypeStr=uint8  SaturateOnIntegerOverflow=on
  Gain1 : Gain  Gain=2  OutDataTypeStr=uint8  SaturateOnIntegerOverflow=on
  Gain2 : Gain  Gain=4  OutDataTypeStr=uint8  SaturateOnIntegerOverflow=on
  Gain3 : Gain  Gain=8  OutDataTypeStr=uint8  SaturateOnIntegerOverflow=on
  Out1 : Outport
  wires:
  Cruise Enable/1 -> Data Type Conversion/1
  Cruise Active/1 -> Data Type Conversion1/1
  Fault Ack/1 -> Data Type Conversion2/1
  Add/1 -> Out1/1
  Gain/1 -> Add/1
  Gain1/1 -> Add/2
  Gain2/1 -> Add/3
  Data Type Conversion/1 -> Gain/1
  Data Type Conversion1/1 -> Gain1/1
  Data Type Conversion2/1 -> Gain2/1
  Data Type Conversion3/1 -> Gain3/1
  Utility 1/1 -> Data Type Conversion3/1
  Gain3/1 -> Add/4

== system p1_MCU/Steering Control/Steering Controller ==
  Driver Input : Inport
  Steering Addition : Inport  Port=2
  Ackermann Correction : Subsystem
  Add : Sum
  Bus Selector1 : BusSelector  OutputSignals=HW Primary
  Bus Selector4 : BusSelector  OutputSignals=Utility 1
  D2R : Gain  Gain=pi/180  SaturateOnIntegerOverflow=on  OutDataTypeStr=Inherit: Same as input  ParamDataTypeStr=Inherit: Same as input
  Data Store Memory : DataStoreMemory  DataStoreName=Toe_Offset  ReadBeforeWriteMsg=warning  WriteAfterWriteMsg=warning  WriteAfterReadMsg=warning  ShowAdditionalParam=off  OutDataTypeStr=double
  Data Store Read : DataStoreRead  DataStoreName=Toe_Offset  IndexOptions=Index vector (dialog)  Indices=1  OutputSizes=1
  HAL-9000 : Subsystem  mask{enabled=off, maneuver=Chirp, amplitude=5, delay=0, duration=20, startfreq=.5, endfreq=5}
      mask prompts: enabled "Enable HAL-9000 Automated Steering Maneuver System"; maneuver "Steering manuever"; amplitude "Amplitude (deg)"; delay "Delay (sec)"; duration "Duration (sec)"; startfreq "Initial frequency (Hz)"; endfreq "Final frequency (Hz)"
      mask init:
      | switch(maneuver)
      | 	case 'Step'
      | 		maneuver=1;
      | 	case 'Ramp'
      | 		maneuver=2;
      | 	case 'Chirp'
      | 		maneuver=3;
      | 	case 'Double-step'
      | 		maneuver=4;
      | 	case 'Double chirp'
      | 		maneuver=5;
      | end
      | switch(enabled)
      | 	case 'on'
      | 		enabled=1;
      | 	case 'off'
      | 		enabled=0;
      | end
      mask Callback enabled:
      | if(strcmp(get_param(gcb,'enabled'),'off'))
      | 	set_param(gcb,'MaskEnables',{'on','off','off','off','off','off','off'});
      | else
      | 	set_param(gcb,'MaskEnables',{'on','on','on','on','on','on','on'});
      | end
      mask TypeOptions maneuver: Step | Ramp | Chirp | Double step | Double chirp
      mask Callback maneuver:
      | switch(get_param(gcb,'maneuver'))
      | 	case 'Step'
      | 		set_param(gcb,'MaskVisibilities',{'on','on','on','on','off','off','off'});
      | 	case 'Double step'
      | 		set_param(gcb,'MaskVisibilities',{'on','on','on','on','on','off','off'});
      | 	case 'Ramp'
      | 		set_param(gcb,'MaskVisibilities',{'on','on','on','on','on','off','off'});
      | 	case 'Chirp'
      | 		set_param(gcb,'MaskVisibilities',{'on','on','on','on','on','on','on'});
      | 	case 'Double chirp'
      | 		set_param(gcb,'MaskVisibilities',{'on','on','on','on','on','on','on'});
      | end
  Heavy Filter : DiscreteFilter  Numerator=[1*(2*pi*Ts_MCU)]  Denominator=[1 1*(2*pi*Ts_MCU)-1]  SampleTime=Ts_MCU
  Input Selector : Constant
  Multiport Switch : MultiPortSwitch  SaturateOnIntegerOverflow=off  InputSameDT=off
  Mux1 : Mux  Inputs=2
  Nominal Filter : DiscreteFilter  Numerator=[wc*2*pi*Ts_MCU]  Denominator=[1 wc*2*pi*Ts_MCU-1]  SampleTime=Ts_MCU
  Software Steering Limit : Saturate  UpperLimit=steering_limit*sr*pi/180  LowerLimit=-steering_limit*sr*pi/180
  Software Steering Limit1 : Saturate  UpperLimit=steering_limit*pi/180  LowerLimit=-steering_limit*pi/180
  Steering Ratio1 : Gain  Gain=sr  SaturateOnIntegerOverflow=on  OutDataTypeStr=Inherit: Same as input  ParamDataTypeStr=Inherit: Same as input
  Steering Ratio : Gain  Gain=1/sr  SaturateOnIntegerOverflow=on  OutDataTypeStr=Inherit: Same as input  ParamDataTypeStr=Inherit: Same as input
  Subtract : Sum  Inputs=-+
  Sum : Sum  Inputs=++|
  Sum1 : Sum  Inputs=+++
  Switch : Switch  Criteria=u2 ~= 0  Threshold=0.5  SaturateOnIntegerOverflow=off  InputSameDT=off
  Steering Angle Commands : Outport
  wires:
  Data Store Read/1 -> D2R/1
  D2R/1 -> Subtract/1, Add/1
  Mux1/1 -> Steering Angle Commands/1
  Sum1/1 -> Switch/1
  Switch/1 -> Multiport Switch/4
  Input Selector/1 -> Multiport Switch/1
  HAL-9000/1(Offset) -> Sum1/3
  Heavy Filter/1 -> Sum1/2
  Sum/1 -> Multiport Switch/3
  Nominal Filter/1 -> Switch/3, Multiport Switch/2, Software Steering Limit/1
  Steering Ratio1/1 -> Sum1/1, Sum/2
  Steering Addition/1 -> Steering Ratio1/1
  Bus Selector4/1 -> Switch/2, HAL-9000/1(Trigger)  "<Utility 1>"
  Multiport Switch/1 -> Steering Ratio/1
  Software Steering Limit/1 -> Sum/1
  Software Steering Limit1/1 -> Ackermann Correction/1(Ackermann Angle)
  Steering Ratio/1 -> Software Steering Limit1/1
  Ackermann Correction/1(L Steer Angle) -> Subtract/2
  Ackermann Correction/2(R Steer Angle) -> Add/2
  Subtract/1 -> Mux1/1
  Add/1 -> Mux1/2
  Bus Selector1/1 -> Heavy Filter/1, Nominal Filter/1  "<HW Primary>"
  Driver Input/1 -> Bus Selector4/1, Bus Selector1/1
